simulink model "Model_design"  (R2021a)
settings: Solver=VariableStepAuto  StartTime=0.0  StopTime=10.0  RelTol=1e-3
undefined symbols (not defined in the file): chi_c, k_d_phi, k_i_chi, k_p_chi, k_p_phi, MAV
settings Model: Creator=DELL  LastModifiedBy=DELL

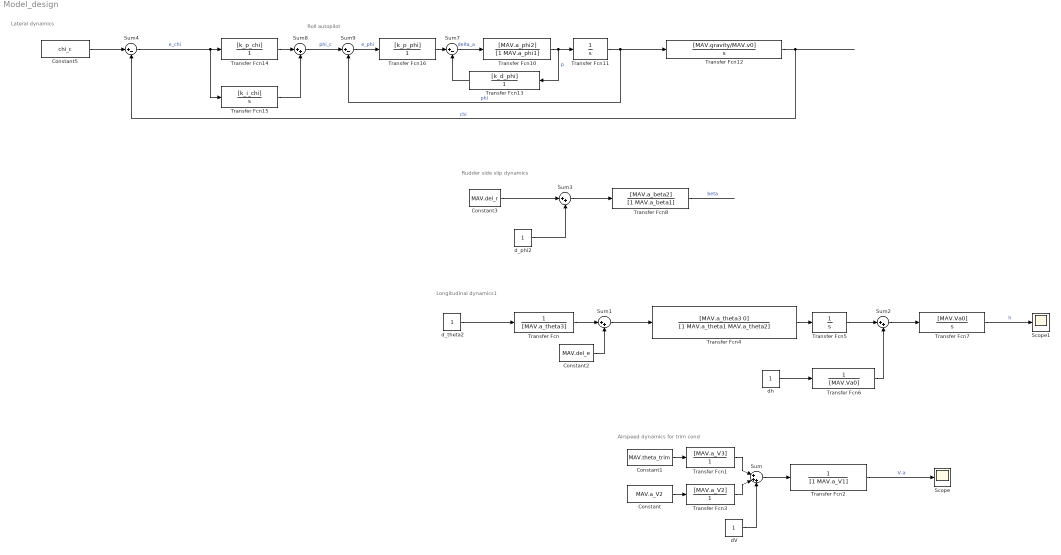
== system Model_design ==
  note: Roll autopilot
  note: Lateral dynamics
  note: Airspeed dynamics for trim cond
  note: Longitudinal dynamics1
  note: Rudder side slip dynamics
  Constant : Constant  Value=MAV.a_V2
  Constant1 : Constant  Value=MAV.theta_trim
  Constant2 : Constant  Value=MAV.del_e
  Constant3 : Constant  Value=MAV.del_r
  Constant5 : Constant  Value=chi_c
  Scope : Scope
  Scope1 : Scope
  Sum : Sum  Inputs=|+++
  Sum{1..3,8} (4 alike) : Sum  Inputs=|++
  Sum4 : Sum  Inputs=|+-
  Sum7 : Sum  Inputs=|+-
  Sum9 : Sum  Inputs=|+-
  Transfer Fcn : TransferFcn  Denominator=[MAV.a_theta3]
  Transfer Fcn1 : TransferFcn  Numerator=[MAV.a_V3]  Denominator=[1]
  Transfer Fcn10 : TransferFcn  Numerator=[MAV.a_phi2]  Denominator=[1 MAV.a_phi1]
  Transfer Fcn11 : TransferFcn  Denominator=[1 0]
  Transfer Fcn12 : TransferFcn  Numerator=[MAV.gravity/MAV.v0]  Denominator=[1 0]
  Transfer Fcn13 : TransferFcn  Numerator=[k_d_phi]  Denominator=[1]
  Transfer Fcn14 : TransferFcn  Numerator=[k_p_chi]  Denominator=1
  Transfer Fcn15 : TransferFcn  Numerator=[k_i_chi]  Denominator=[1 0]
  Transfer Fcn16 : TransferFcn  Numerator=[k_p_phi]  Denominator=1
  Transfer Fcn2 : TransferFcn  Denominator=[1 MAV.a_V1]
  Transfer Fcn3 : TransferFcn  Numerator=[MAV.a_V2]  Denominator=[1]
  Transfer Fcn4 : TransferFcn  Numerator=[MAV.a_theta3 0]  Denominator=[1 MAV.a_theta1 MAV.a_theta2]
  Transfer Fcn5 : TransferFcn  Denominator=[1 0]
  Transfer Fcn6 : TransferFcn  Denominator=[MAV.Va0]
  Transfer Fcn7 : TransferFcn  Numerator=[MAV.Va0]  Denominator=[1 0]
  Transfer Fcn8 : TransferFcn  Numerator=[MAV.a_beta2]  Denominator=[1 MAV.a_beta1]
  dV : Constant
  d_phi2 : Constant
  d_theta2 : Constant
  dh : Constant
  wires:
  Sum3/1 -> Transfer Fcn8/1
  Transfer Fcn12/1 -> Sum4/2  "chi"
  Transfer Fcn7/1 -> Scope1/1  "h"
  Transfer Fcn2/1 -> Scope/1  "V-a"
  Sum/1 -> Transfer Fcn2/1
  Constant1/1 -> Transfer Fcn1/1
  Transfer Fcn8/1 -> ?  "beta"
  Transfer Fcn3/1 -> Sum/2
  dV/1 -> Sum/3
  Transfer Fcn1/1 -> Sum/1
  Transfer Fcn5/1 -> Sum2/1
  Constant/1 -> Transfer Fcn3/1
  Sum1/1 -> Transfer Fcn4/1
  Transfer Fcn4/1 -> Transfer Fcn5/1
  Transfer Fcn6/1 -> Sum2/2
  Constant2/1 -> Sum1/2
  Constant3/1 -> Sum3/1
  dh/1 -> Transfer Fcn6/1
  d_phi2/1 -> Sum3/2
  d_theta2/1 -> Transfer Fcn/1
  Sum2/1 -> Transfer Fcn7/1
  Transfer Fcn/1 -> Sum1/1
  Transfer Fcn14/1 -> Sum8/1
  Transfer Fcn15/1 -> Sum8/2
  Constant5/1 -> Sum4/1
  Sum4/1 -> Transfer Fcn15/1, Transfer Fcn14/1  "e_chi"
  Transfer Fcn16/1 -> Sum7/1
  Sum8/1 -> Sum9/1  "phi_c"
  Transfer Fcn11/1 -> Transfer Fcn12/1, Sum9/2  "phi"
  Sum7/1 -> Transfer Fcn10/1  "delta_a"
  Transfer Fcn10/1 -> Transfer Fcn13/1, Transfer Fcn11/1  "p"
  Transfer Fcn13/1 -> Sum7/2
  Sum9/1 -> Transfer Fcn16/1  "e_phi"
